simulink model "FINAL_FULL_CONTROLLER"  (R2023b)
settings: Solver=VariableStepAuto  StartTime=0.0  StopTime=10  MaxStep=1e-2  RelTol=1e-6
values from neighbouring files (symbols this model uses):
  cq = -rho*(pi*re^2)*(re^2)*Cq    (= -5.82688103164e-07)    [PARAMETRI_DRONE.m]
  Cq = 0.002508    [PARAMETRI_DRONE.m]
  ct = rho*(pi*re^2)*(re^2)*Ct    (= 3.66666014519e-06)    [PARAMETRI_DRONE.m]
  Ct = 0.015782    [PARAMETRI_DRONE.m]
  dx = 0.035/(2*sqrt(2))    [PARAMETRI_DRONE.m]
  dy = 0.035/(2*sqrt(2))    [PARAMETRI_DRONE.m]
  g = 9.81    [PARAMETRI_DRONE.m]
  I = Inertial_Matrix_DART(m1, m2, m3, m4, m, d1, d2, d3, d4, d5, dx, dy, r, h, a1, b1, c1, a2, b2, c2, a3, b3, c3, a4, b4, c4)    [PARAMETRI_DRONE.m]
  m = 0.055    [PARAMETRI_DRONE.m]
  m1 = 0.135    [PARAMETRI_DRONE.m]
  m2 = 0.602    [PARAMETRI_DRONE.m]
  m3 = 0.228    [PARAMETRI_DRONE.m]
  m4 = 0.055    [PARAMETRI_DRONE.m]
  re = 0.0889    [PARAMETRI_DRONE.m]
  wmax = RPMmax*(2*pi)/60    (= 2350.85378268)    [PARAMETRI_DRONE.m]
libraries: slpidlib x9, simulink x4, shared6dof x1, aerolibpropulsion2 x1, dspinverses x1
(part 1 of 2)
settings Model: Creator=elisa  LastModifiedBy=elisa
settings DebuggingCC: ParameterOverflowMsg=none  ParameterUnderflowMsg=error

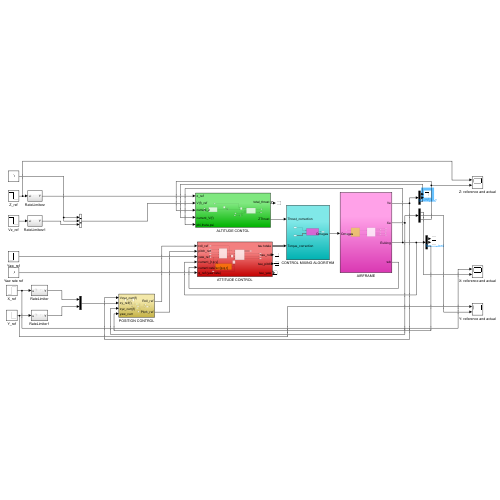
[thumbnail: Simulink's stored preview of the top-level diagram]
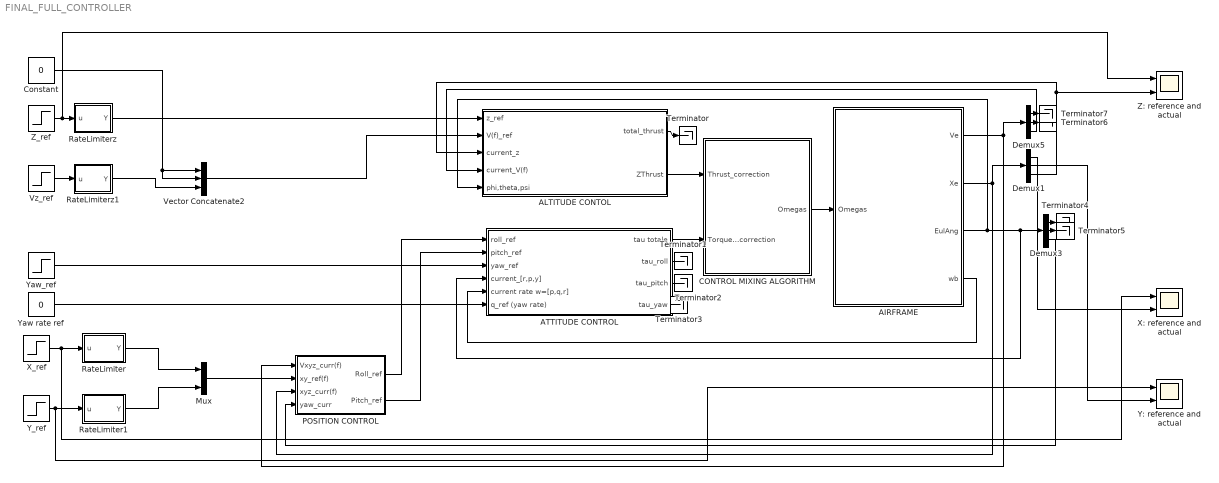
== system FINAL_FULL_CONTROLLER ==
  AIRFRAME : Subsystem
  ALTITUDE CONTOL : Subsystem
  ATTITUDE CONTROL : Subsystem
  CONTROL MIXING ALGORITHM : Subsystem
  Constant : Constant  Value=0
  Demux1 : Demux  Outputs=3
  Demux3 : Demux  Outputs=3
  Demux5 : Demux  Outputs=3
  Mux : Mux  Inputs=2
  POSITION CONTROL : Subsystem
  RateLimiter : Subsystem
  RateLimiter1 : Subsystem
  RateLimiterz : Subsystem
  RateLimiterz1 : Subsystem
  Terminator{,1..7} (8 alike) : Terminator
  Vector Concatenate2 : Concatenate  NumInputs=3
  Vz_ref : Step  After=-1  SampleTime=0
  X: reference and actual : Scope  NumInputPorts=2
  X_ref : Step  Time=2  After=0.5  SampleTime=0
  Y: reference and actual : Scope  NumInputPorts=2
  Y_ref : Step  Time=5  After=-0.2  SampleTime=0
  Yaw rate ref : Constant  Value=0
  Yaw_ref : Step  Time=6  After=pi/4  SampleTime=0
  Z: reference and actual : Scope  NumInputPorts=2
  Z_ref : Step  After=-1  SampleTime=0
  wires:
  Yaw_ref/1 -> ATTITUDE CONTROL/3(yaw_ref)
  Constant/1 -> Vector Concatenate2/1, Vector Concatenate2/2
  Yaw rate ref/1 -> ATTITUDE CONTROL/6(q_ref (yaw rate))
  AIRFRAME/4(wb) -> ATTITUDE CONTROL/5(current rate w=[p,q,r])
  AIRFRAME/2(Xe) -> POSITION CONTROL/3(xyz_curr(f)), Demux1/1
  ALTITUDE CONTOL/2(ZThrust) -> CONTROL MIXING ALGORITHM/1(Thrust_correction)
  ATTITUDE CONTROL/1(tau totale) -> CONTROL MIXING ALGORITHM/2(Torque_correction)
  Demux3/3 -> POSITION CONTROL/4(yaw_curr)
  AIRFRAME/1(Ve) -> POSITION CONTROL/1(Vxyz_curr(f)), Demux5/1
  POSITION CONTROL/1(Roll_ref) -> ATTITUDE CONTROL/1(roll_ref)
  X_ref/1 -> X: reference and actual/1, RateLimiter/1(u)
  RateLimiter/1(Y) -> Mux/1
  Y_ref/1 -> Y: reference and actual/1, RateLimiter1/1(u)
  RateLimiter1/1(Y) -> Mux/2
  Z_ref/1 -> Z: reference and actual/1, RateLimiterz/1(u)
  Vz_ref/1 -> RateLimiterz1/1(u)
  RateLimiterz1/1(Y) -> Vector Concatenate2/3
  RateLimiterz/1(Y) -> ALTITUDE CONTOL/1(z_ref)
  Vector Concatenate2/1 -> ALTITUDE CONTOL/2(V(f)_ref)
  Demux1/3 -> ALTITUDE CONTOL/3(current_z), Z: reference and actual/2
  Demux5/3 -> ALTITUDE CONTOL/4(current_V(f))
  AIRFRAME/3(EulAng) -> Demux3/1, ATTITUDE CONTROL/4(current_[r,p,y]), ALTITUDE CONTOL/5(phi,theta,psi)
  Mux/1 -> POSITION CONTROL/2(xy_ref(f))
  POSITION CONTROL/2(Pitch_ref) -> ATTITUDE CONTROL/2(pitch_ref)
  ATTITUDE CONTROL/2(tau_roll) -> Terminator1/1
  ATTITUDE CONTROL/3(tau_pitch) -> Terminator2/1
  ALTITUDE CONTOL/1(total_thrust) -> Terminator/1
  CONTROL MIXING ALGORITHM/1(Omegas) -> AIRFRAME/1(Omegas)
  Demux1/1 -> X: reference and actual/2
  Demux1/2 -> Y: reference and actual/2
  Demux3/1 -> Terminator4/1
  Demux3/2 -> Terminator5/1
  Demux5/2 -> Terminator6/1
  Demux5/1 -> Terminator7/1

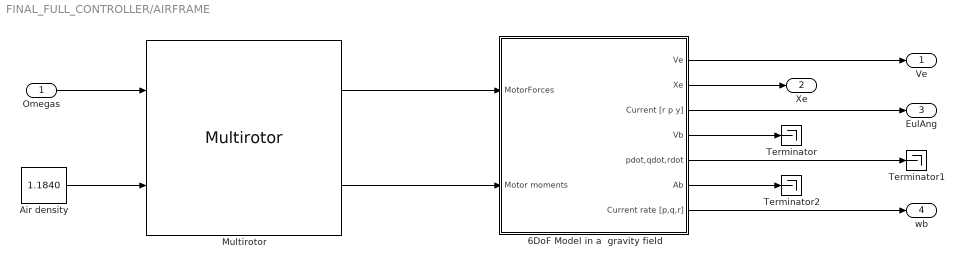
== system FINAL_FULL_CONTROLLER/AIRFRAME ==
  Omegas : Inport
  6DoF Model in a  gravity field : Subsystem
  Air density : Constant  Value=1.1840
  Multirotor : aerolibpropulsion2/Multirotor  units=Metric (MKS)  modelMode=Without flap effects  blockSelect=Multiple  config=Quadcopter X  Nr=4  l=sqrt(2)*dx  h=h  Arm=[0.0441234631460406 0.0441234631460406 -0.0441234631460406 -0.0441234631460406;-0.0441234631460406 0.0441234631460406 0.0441234631460406 -0.0441234631460406;-0.0159 -0.0159 -0.0159 -0.0159]  Nb=2  CTcheck=off  CT=Ct  CQ=Cq  CTout=off  R=re  c=0.0080  e=0  clalpha=5.5  gamma=0.6051  twistType=Linear  theta0=0.2548  theta1=-0.1361  thetaTip=0.1018  Vb=[0;0;0]  pqr=[0;0;0]
      settings: LibrarySourceBlock=aerolibrotor/Rotor
  Terminator : Terminator
  Terminator1 : Terminator
  Terminator2 : Terminator
  Ve : Outport
  Xe : Outport  Port=2
  EulAng : Outport  Port=3
  wb : Outport  Port=4
  wires:
  6DoF Model in a  gravity field/4(Vb) -> Terminator/1
  6DoF Model in a  gravity field/6(Ab) -> Terminator2/1
  6DoF Model in a  gravity field/5(pdot,qdot,rdot) -> Terminator1/1
  6DoF Model in a  gravity field/1(Ve) -> Ve/1
  6DoF Model in a  gravity field/2(Xe) -> Xe/1
  6DoF Model in a  gravity field/3(Current [r p y]) -> EulAng/1
  6DoF Model in a  gravity field/7(Current rate [p,q,r]) -> wb/1
  Multirotor/1 -> 6DoF Model in a  gravity field/1(MotorForces)
  Multirotor/2 -> 6DoF Model in a  gravity field/2(Motor moments)
  Omegas/1 -> Multirotor/1
  Air density/1 -> Multirotor/2

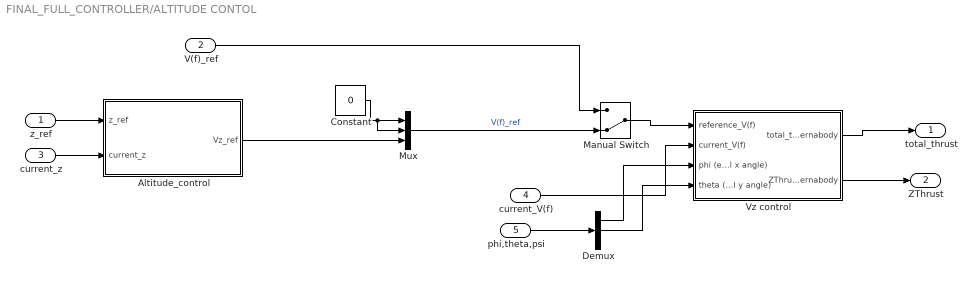
== system FINAL_FULL_CONTROLLER/ALTITUDE CONTOL ==
  z_ref : Inport
  V(f)_ref : Inport  Port=2
  current_z : Inport  Port=3
  current_V(f) : Inport  Port=4
  phi,theta,psi : Inport  Port=5
  Altitude_control : Subsystem
  Constant : Constant  Value=0
  Demux : Demux  Outputs=3
  Manual Switch : ManualSwitch  CurrentSetting=0
  Mux : Mux  Inputs=3
  Vz control : Subsystem
  total_thrust : Outport
  ZThrust : Outport  Port=2
  wires:
  current_V(f)/1 -> Vz control/2(current_V(f))
  z_ref/1 -> Altitude_control/1(z_ref)
  current_z/1 -> Altitude_control/2(current_z)
  Manual Switch/1 -> Vz control/1(reference_V(f))
  Vz control/1(total_thrust_ternabody) -> total_thrust/1
  Vz control/2(ZThrust_ternabody) -> ZThrust/1
  Mux/1 -> Manual Switch/2  "V(f)_ref"
  Altitude_control/1(Vz_ref) -> Mux/3
  Constant/1 -> Mux/2, Mux/1
  V(f)_ref/1 -> Manual Switch/1
  phi,theta,psi/1 -> Demux/1
  Demux/1 -> Vz control/3(phi (eul x angle))
  Demux/2 -> Vz control/4(theta (eul y angle))

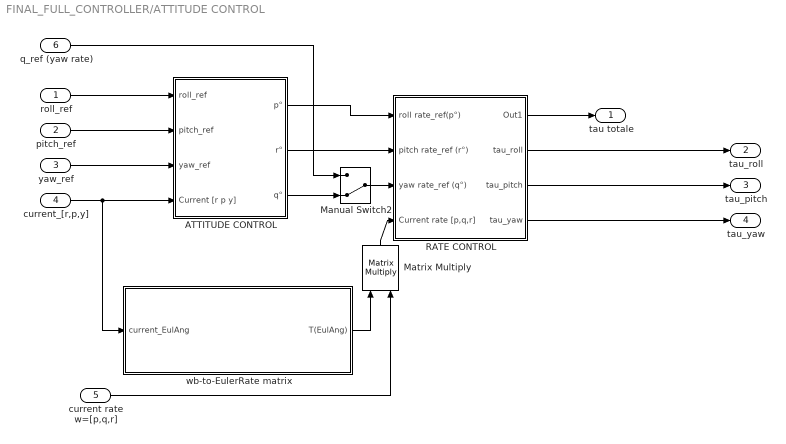
== system FINAL_FULL_CONTROLLER/ATTITUDE CONTROL ==
  roll_ref : Inport
  pitch_ref : Inport  Port=2
  yaw_ref : Inport  Port=3
  current_[r,p,y] : Inport  Port=4
  current rate w=[p,q,r] : Inport  Port=5
  q_ref (yaw rate) : Inport  Port=6
  ATTITUDE CONTROL : Subsystem
  Manual Switch2 : ManualSwitch  CurrentSetting=0
  Matrix Multiply : Product  Multiplication=Matrix(*)
  RATE CONTROL : Subsystem
  wb-to-EulerRate matrix : Subsystem
  tau totale : Outport
  tau_roll : Outport  Port=2
  tau_pitch : Outport  Port=3
  tau_yaw : Outport  Port=4
  wires:
  pitch_ref/1 -> ATTITUDE CONTROL/2(pitch_ref)
  roll_ref/1 -> ATTITUDE CONTROL/1(roll_ref)
  yaw_ref/1 -> ATTITUDE CONTROL/3(yaw_ref)
  current_[r,p,y]/1 -> wb-to-EulerRate matrix/1(current_EulAng), ATTITUDE CONTROL/4(Current [r p y])
  RATE CONTROL/1(Out1) -> tau totale/1
  ATTITUDE CONTROL/2(r°) -> RATE CONTROL/2(pitch rate_ref (r°))
  Manual Switch2/1 -> RATE CONTROL/3(yaw rate_ref (q°))
  ATTITUDE CONTROL/1(p°) -> RATE CONTROL/1(" roll rate_ref(p°)")
  q_ref (yaw rate)/1 -> Manual Switch2/1
  ATTITUDE CONTROL/3(q°) -> Manual Switch2/2
  RATE CONTROL/3(tau_pitch) -> tau_pitch/1
  RATE CONTROL/4(tau_yaw) -> tau_yaw/1
  RATE CONTROL/2(tau_roll) -> tau_roll/1
  current rate w=[p,q,r]/1 -> Matrix Multiply/2
  wb-to-EulerRate matrix/1(T(EulAng)) -> Matrix Multiply/1
  Matrix Multiply/1 -> RATE CONTROL/4(Current rate [p,q,r])

== system FINAL_FULL_CONTROLLER/CONTROL MIXING ALGORITHM ==
  Thrust_correction : Inport
  Torque_correction : Inport  Port=2
  Control Mixing Algorithm : Subsystem
  Omegas : Outport
  wires:
  Thrust_correction/1 -> Control Mixing Algorithm/1(Thrust)
  Torque_correction/1 -> Control Mixing Algorithm/2(Torque)
  Control Mixing Algorithm/1(Omega_vector) -> Omegas/1

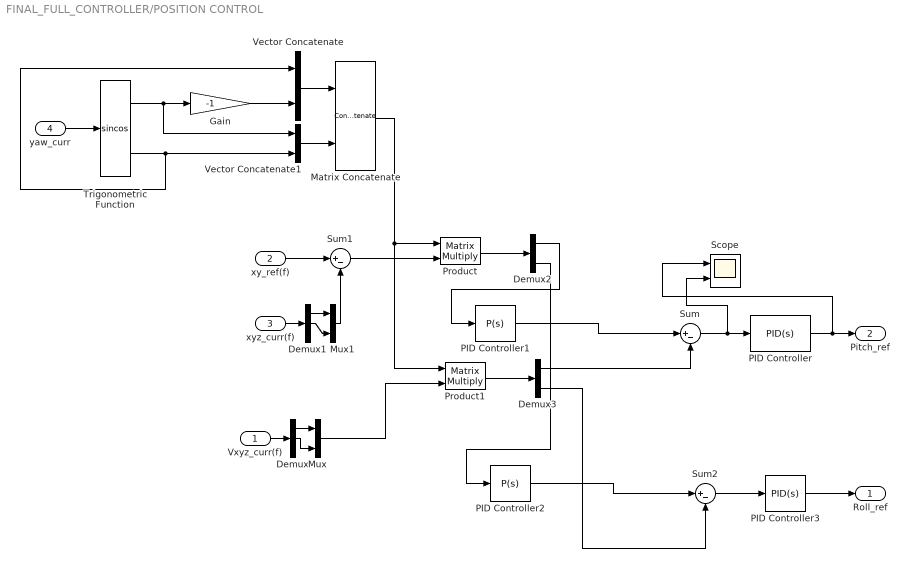
== system FINAL_FULL_CONTROLLER/POSITION CONTROL ==
  Vxyz_curr(f) : Inport
  xy_ref(f) : Inport  Port=2
  xyz_curr(f) : Inport  Port=3
  yaw_curr : Inport  Port=4
  Demux : Demux  Outputs=3
  Demux1 : Demux  Outputs=3
  Demux2 : Demux  Outputs=2
  Demux3 : Demux  Outputs=2
  Gain : Gain  Gain=-1
  Matrix Concatenate : Concatenate  Mode=Multidimensional array  ConcatenateDimension=2
  Mux : Mux  Inputs=2
  Mux1 : Mux  Inputs=2
  PID Controller : slpidlib/PID Controller  Controller=PID  Form=Parallel  TimeDomain=Continuous-time  UseExternalTs=off  SampleTime=-1  IntegratorMethod=Forward Euler  FilterMethod=Forward Euler  ControllerParametersSource=internal  P=-1.81773619393161  I=-2.23779497117918  UseKiTs=off  D=-0.196003883525991  N=1526.47988950234  UseFilter=on  TunerSelectOption=Transfer Function Based (PID Tuner App)  InitialConditionSource=internal  InitialConditionForIntegrator=0  InitialConditionForFilter=0  DifferentiatorICPrevScaledInput=0  ExternalReset=none  TrackingMode=off  Kt=1  LimitOutput=on  SatLimitsSource=internal  UpperSaturationLimit=pi/4  LowerSaturationLimit=-pi/4  LinearizeAsGain=on  AntiWindupMode=back-calculation  Kb=3  LimitIntegrator=off  UpperIntegratorSaturationLimit=inf  LowerIntegratorSaturationLimit=-inf  POutMin=[]  POutMax=[]  IOutMin=[]  IOutMax=[]  DOutMin=[]  DOutMax=[]  NOutMin=[]  NOutMax=[]  SumOutMin=[]  SumOutMax=[]  SaturationOutMin=[]  SaturationOutMax=[]  PParamMin=[]  PParamMax=[]  IParamMin=[]  IParamMax=[]  DParamMin=[]  DParamMax=[]  NParamMin=[]  NParamMax=[]  KbParamMin=[]  KbParamMax=[]  KtParamMin=[]  KtParamMax=[]  KbOutMin=[]  KbOutMax=[]  KtOutMin=[]  KtOutMax=[]  IntegratorOutMin=[]  IntegratorOutMax=[]  FilterOutMin=[]  FilterOutMax=[]  SumI1OutMin=[]  SumI1OutMax=[]  SumI2OutMin=[]  SumI2OutMax=[]  SumI3OutMin=[]  SumI3OutMax=[]  SumI4OutMin=[]  SumI4OutMax=[]  SumDOutMin=[]  SumDOutMax=[]  DifferentiatorOutMin=[]  DifferentiatorOutMax=[]  FilterDiffOutCoefMin=[]  FilterDiffOutCoefMax=[]  ReciprocalOutMin=[]  ReciprocalOutMax=[]  SumDenOutMin=[]  SumDenOutMax=[]  SumNumOutMin=[]  SumNumOutMax=[]  DivideOutMin=[]  DivideOutMax=[]  UdiffTsProdOutMin=[]  UdiffTsProdOutMax=[]  NTsProdOutMin=[]  NTsProdOutMax=[]  UintegralTsProdOutMin=[]  UintegralTsProdOutMax=[]  UngainTsProdOutMin=[]  UngainTsProdOutMax=[]  ClampingZeroOutDataTypeStr=Inherit: Inherit via back propagation  ClampingZeroOutMin=[]  ClampingZeroOutMax=[]  FilterDenConstantOutDataTypeStr=Inherit: Inherit via back propagation  FilterDenConstantOutMin=[]  FilterDenConstantOutMax=[]  PCopyOutDataTypeStr=Inherit: Inherit via back propagation  PCopyOutMin=[]  PCopyOutMax=[]  NCopyOutDataTypeStr=Inherit: Inherit via back propagation  NCopyOutMin=[]  NCopyOutMax=[]  IntegratorContinuousStateAttributes=''  IntegratorStateMustResolveToSignalObject=off  IntegratorRTWStateStorageClass=Auto  FilterContinuousStateAttributes=''  FilterStateMustResolveToSignalObject=off  FilterRTWStateStorageClass=Auto  ParallelPVariant=InternalParameters  IdealPVariant=Disabled  IVariant=InternalParameters  DVariant=InternalParameters  IntegratorVariant=Continuous  SatVariant=Enabled  AWVariant=BackCalculation  PCopyVariant=Disabled  TRVariant=Disabled  FdbkBlocksVariant=Forward  IdealPFdbkVariant=Disabled  SatFdbkVariant=Disabled  DerivativeFilterVariant=ContFilter  NVariant=InternalParameters  NCopyVariant=Disabled  FilterICVariant=InternalICsFilter  IntegratorICVariant=InternalICs  ExternalResetVariant=Disabled  TRSumVariant=Passthrough  SumFdbkVariant=Disabled  SumVariant=Sum_PID  TsampFilterVariant=InternalTs  TsampNgainVariant=Passthrough  TsampIntegralVariant=Disabled_SignalSpec  ExternalSaturationOutDataTypeStr=Inherit: Same as second input
  PID Controller1 : slpidlib/PID Controller  Controller=P  Form=Parallel  TimeDomain=Continuous-time  UseExternalTs=off  SampleTime=-1  IntegratorMethod=Forward Euler  FilterMethod=Forward Euler  ControllerParametersSource=internal  P=6.73453826135935  I=1  UseKiTs=off  D=0  N=100  UseFilter=on  TunerSelectOption=Transfer Function Based (PID Tuner App)  InitialConditionSource=internal  InitialConditionForIntegrator=0  InitialConditionForFilter=0  DifferentiatorICPrevScaledInput=0  ExternalReset=none  TrackingMode=off  Kt=1  LimitOutput=off  SatLimitsSource=internal  UpperSaturationLimit=inf  LowerSaturationLimit=-inf  LinearizeAsGain=on  AntiWindupMode=none  Kb=1  LimitIntegrator=off  UpperIntegratorSaturationLimit=inf  LowerIntegratorSaturationLimit=-inf  POutMin=[]  POutMax=[]  IOutMin=[]  IOutMax=[]  DOutMin=[]  DOutMax=[]  NOutMin=[]  NOutMax=[]  SumOutMin=[]  SumOutMax=[]  SaturationOutMin=[]  SaturationOutMax=[]  PParamMin=[]  PParamMax=[]  IParamMin=[]  IParamMax=[]  DParamMin=[]  DParamMax=[]  NParamMin=[]  NParamMax=[]  KbParamMin=[]  KbParamMax=[]  KtParamMin=[]  KtParamMax=[]  KbOutMin=[]  KbOutMax=[]  KtOutMin=[]  KtOutMax=[]  IntegratorOutMin=[]  IntegratorOutMax=[]  FilterOutMin=[]  FilterOutMax=[]  SumI1OutMin=[]  SumI1OutMax=[]  SumI2OutMin=[]  SumI2OutMax=[]  SumI3OutMin=[]  SumI3OutMax=[]  SumI4OutMin=[]  SumI4OutMax=[]  SumDOutMin=[]  SumDOutMax=[]  DifferentiatorOutMin=[]  DifferentiatorOutMax=[]  FilterDiffOutCoefMin=[]  FilterDiffOutCoefMax=[]  ReciprocalOutMin=[]  ReciprocalOutMax=[]  SumDenOutMin=[]  SumDenOutMax=[]  SumNumOutMin=[]  SumNumOutMax=[]  DivideOutMin=[]  DivideOutMax=[]  UdiffTsProdOutMin=[]  UdiffTsProdOutMax=[]  NTsProdOutMin=[]  NTsProdOutMax=[]  UintegralTsProdOutMin=[]  UintegralTsProdOutMax=[]  UngainTsProdOutMin=[]  UngainTsProdOutMax=[]  ClampingZeroOutDataTypeStr=Inherit: Inherit via back propagation  ClampingZeroOutMin=[]  ClampingZeroOutMax=[]  FilterDenConstantOutDataTypeStr=Inherit: Inherit via back propagation  FilterDenConstantOutMin=[]  FilterDenConstantOutMax=[]  PCopyOutDataTypeStr=Inherit: Inherit via back propagation  PCopyOutMin=[]  PCopyOutMax=[]  NCopyOutDataTypeStr=Inherit: Inherit via back propagation  NCopyOutMin=[]  NCopyOutMax=[]  IntegratorContinuousStateAttributes=''  IntegratorStateMustResolveToSignalObject=off  IntegratorRTWStateStorageClass=Auto  FilterContinuousStateAttributes=''  FilterStateMustResolveToSignalObject=off  FilterRTWStateStorageClass=Auto  ParallelPVariant=InternalParameters  IdealPVariant=Disabled  IVariant=Disabled  DVariant=Disabled  IntegratorVariant=Disabled  SatVariant=Disabled  AWVariant=Disabled  PCopyVariant=Disabled  TRVariant=Disabled  FdbkBlocksVariant=Forward  IdealPFdbkVariant=Disabled  SatFdbkVariant=Disabled  DerivativeFilterVariant=Disabled  NVariant=Disabled  NCopyVariant=Disabled_SignalSpec  FilterICVariant=Disabled  IntegratorICVariant=Disabled  ExternalResetVariant=Disabled  TRSumVariant=Passthrough  SumFdbkVariant=Disabled  SumVariant=Passthrough_P  TsampFilterVariant=InternalTs  TsampNgainVariant=Passthrough  TsampIntegralVariant=Disabled_SignalSpec  ExternalSaturationOutDataTypeStr=Inherit: Same as second input
  PID Controller2 : slpidlib/PID Controller  Controller=P  Form=Parallel  TimeDomain=Continuous-time  UseExternalTs=off  SampleTime=-1  IntegratorMethod=Forward Euler  FilterMethod=Forward Euler  ControllerParametersSource=internal  P=6.91764423663116  I=1  UseKiTs=off  D=0  N=100  UseFilter=on  TunerSelectOption=Transfer Function Based (PID Tuner App)  InitialConditionSource=internal  InitialConditionForIntegrator=0  InitialConditionForFilter=0  DifferentiatorICPrevScaledInput=0  ExternalReset=none  TrackingMode=off  Kt=1  LimitOutput=off  SatLimitsSource=internal  UpperSaturationLimit=inf  LowerSaturationLimit=-inf  LinearizeAsGain=on  AntiWindupMode=none  Kb=1  LimitIntegrator=off  UpperIntegratorSaturationLimit=inf  LowerIntegratorSaturationLimit=-inf  POutMin=[]  POutMax=[]  IOutMin=[]  IOutMax=[]  DOutMin=[]  DOutMax=[]  NOutMin=[]  NOutMax=[]  SumOutMin=[]  SumOutMax=[]  SaturationOutMin=[]  SaturationOutMax=[]  PParamMin=[]  PParamMax=[]  IParamMin=[]  IParamMax=[]  DParamMin=[]  DParamMax=[]  NParamMin=[]  NParamMax=[]  KbParamMin=[]  KbParamMax=[]  KtParamMin=[]  KtParamMax=[]  KbOutMin=[]  KbOutMax=[]  KtOutMin=[]  KtOutMax=[]  IntegratorOutMin=[]  IntegratorOutMax=[]  FilterOutMin=[]  FilterOutMax=[]  SumI1OutMin=[]  SumI1OutMax=[]  SumI2OutMin=[]  SumI2OutMax=[]  SumI3OutMin=[]  SumI3OutMax=[]  SumI4OutMin=[]  SumI4OutMax=[]  SumDOutMin=[]  SumDOutMax=[]  DifferentiatorOutMin=[]  DifferentiatorOutMax=[]  FilterDiffOutCoefMin=[]  FilterDiffOutCoefMax=[]  ReciprocalOutMin=[]  ReciprocalOutMax=[]  SumDenOutMin=[]  SumDenOutMax=[]  SumNumOutMin=[]  SumNumOutMax=[]  DivideOutMin=[]  DivideOutMax=[]  UdiffTsProdOutMin=[]  UdiffTsProdOutMax=[]  NTsProdOutMin=[]  NTsProdOutMax=[]  UintegralTsProdOutMin=[]  UintegralTsProdOutMax=[]  UngainTsProdOutMin=[]  UngainTsProdOutMax=[]  ClampingZeroOutDataTypeStr=Inherit: Inherit via back propagation  ClampingZeroOutMin=[]  ClampingZeroOutMax=[]  FilterDenConstantOutDataTypeStr=Inherit: Inherit via back propagation  FilterDenConstantOutMin=[]  FilterDenConstantOutMax=[]  PCopyOutDataTypeStr=Inherit: Inherit via back propagation  PCopyOutMin=[]  PCopyOutMax=[]  NCopyOutDataTypeStr=Inherit: Inherit via back propagation  NCopyOutMin=[]  NCopyOutMax=[]  IntegratorContinuousStateAttributes=''  IntegratorStateMustResolveToSignalObject=off  IntegratorRTWStateStorageClass=Auto  FilterContinuousStateAttributes=''  FilterStateMustResolveToSignalObject=off  FilterRTWStateStorageClass=Auto  ParallelPVariant=InternalParameters  IdealPVariant=Disabled  IVariant=Disabled  DVariant=Disabled  IntegratorVariant=Disabled  SatVariant=Disabled  AWVariant=Disabled  PCopyVariant=Disabled  TRVariant=Disabled  FdbkBlocksVariant=Forward  IdealPFdbkVariant=Disabled  SatFdbkVariant=Disabled  DerivativeFilterVariant=Disabled  NVariant=Disabled  NCopyVariant=Disabled_SignalSpec  FilterICVariant=Disabled  IntegratorICVariant=Disabled  ExternalResetVariant=Disabled  TRSumVariant=Passthrough  SumFdbkVariant=Disabled  SumVariant=Passthrough_P  TsampFilterVariant=InternalTs  TsampNgainVariant=Passthrough  TsampIntegralVariant=Disabled_SignalSpec  ExternalSaturationOutDataTypeStr=Inherit: Same as second input
  PID Controller3 : slpidlib/PID Controller  Controller=PID  Form=Parallel  TimeDomain=Continuous-time  UseExternalTs=off  SampleTime=-1  IntegratorMethod=Forward Euler  FilterMethod=Forward Euler  ControllerParametersSource=internal  P=1.72614492788019  I=2.41380700470898  UseKiTs=off  D=0.203044940466474  N=1625.25083963237  UseFilter=on  TunerSelectOption=Transfer Function Based (PID Tuner App)  InitialConditionSource=internal  InitialConditionForIntegrator=0  InitialConditionForFilter=0  DifferentiatorICPrevScaledInput=0  ExternalReset=none  TrackingMode=off  Kt=1  LimitOutput=on  SatLimitsSource=internal  UpperSaturationLimit=pi/4  LowerSaturationLimit=-pi/4  LinearizeAsGain=on  AntiWindupMode=back-calculation  Kb=3  LimitIntegrator=off  UpperIntegratorSaturationLimit=inf  LowerIntegratorSaturationLimit=-inf  POutMin=[]  POutMax=[]  IOutMin=[]  IOutMax=[]  DOutMin=[]  DOutMax=[]  NOutMin=[]  NOutMax=[]  SumOutMin=[]  SumOutMax=[]  SaturationOutMin=[]  SaturationOutMax=[]  PParamMin=[]  PParamMax=[]  IParamMin=[]  IParamMax=[]  DParamMin=[]  DParamMax=[]  NParamMin=[]  NParamMax=[]  KbParamMin=[]  KbParamMax=[]  KtParamMin=[]  KtParamMax=[]  KbOutMin=[]  KbOutMax=[]  KtOutMin=[]  KtOutMax=[]  IntegratorOutMin=[]  IntegratorOutMax=[]  FilterOutMin=[]  FilterOutMax=[]  SumI1OutMin=[]  SumI1OutMax=[]  SumI2OutMin=[]  SumI2OutMax=[]  SumI3OutMin=[]  SumI3OutMax=[]  SumI4OutMin=[]  SumI4OutMax=[]  SumDOutMin=[]  SumDOutMax=[]  DifferentiatorOutMin=[]  DifferentiatorOutMax=[]  FilterDiffOutCoefMin=[]  FilterDiffOutCoefMax=[]  ReciprocalOutMin=[]  ReciprocalOutMax=[]  SumDenOutMin=[]  SumDenOutMax=[]  SumNumOutMin=[]  SumNumOutMax=[]  DivideOutMin=[]  DivideOutMax=[]  UdiffTsProdOutMin=[]  UdiffTsProdOutMax=[]  NTsProdOutMin=[]  NTsProdOutMax=[]  UintegralTsProdOutMin=[]  UintegralTsProdOutMax=[]  UngainTsProdOutMin=[]  UngainTsProdOutMax=[]  ClampingZeroOutDataTypeStr=Inherit: Inherit via back propagation  ClampingZeroOutMin=[]  ClampingZeroOutMax=[]  FilterDenConstantOutDataTypeStr=Inherit: Inherit via back propagation  FilterDenConstantOutMin=[]  FilterDenConstantOutMax=[]  PCopyOutDataTypeStr=Inherit: Inherit via back propagation  PCopyOutMin=[]  PCopyOutMax=[]  NCopyOutDataTypeStr=Inherit: Inherit via back propagation  NCopyOutMin=[]  NCopyOutMax=[]  IntegratorContinuousStateAttributes=''  IntegratorStateMustResolveToSignalObject=off  IntegratorRTWStateStorageClass=Auto  FilterContinuousStateAttributes=''  FilterStateMustResolveToSignalObject=off  FilterRTWStateStorageClass=Auto  ParallelPVariant=InternalParameters  IdealPVariant=Disabled  IVariant=InternalParameters  DVariant=InternalParameters  IntegratorVariant=Continuous  SatVariant=Enabled  AWVariant=BackCalculation  PCopyVariant=Disabled  TRVariant=Disabled  FdbkBlocksVariant=Forward  IdealPFdbkVariant=Disabled  SatFdbkVariant=Disabled  DerivativeFilterVariant=ContFilter  NVariant=InternalParameters  NCopyVariant=Disabled  FilterICVariant=InternalICsFilter  IntegratorICVariant=InternalICs  ExternalResetVariant=Disabled  TRSumVariant=Passthrough  SumFdbkVariant=Disabled  SumVariant=Sum_PID  TsampFilterVariant=InternalTs  TsampNgainVariant=Passthrough  TsampIntegralVariant=Disabled_SignalSpec  ExternalSaturationOutDataTypeStr=Inherit: Same as second input
  Product : Product  Multiplication=Matrix(*)  OutDataTypeStr=single  RndMeth=Zero
  Product1 : Product  Multiplication=Matrix(*)  OutDataTypeStr=single  RndMeth=Zero
  Scope : Scope  NumInputPorts=2
  Sum : Sum  Inputs=|+-
  Sum1 : Sum  Inputs=|+-
  Sum2 : Sum  Inputs=|+-
  Trigonometric Function : Trigonometry  Operator=sincos
  Vector Concatenate : Concatenate
  Vector Concatenate1 : Concatenate
  Roll_ref : Outport
  Pitch_ref : Outport  Port=2
  wires:
  PID Controller/1 -> Scope/1, Pitch_ref/1
  Vxyz_curr(f)/1 -> Demux/1
  xy_ref(f)/1 -> Sum1/1
  xyz_curr(f)/1 -> Demux1/1
  Gain/1 -> Vector Concatenate/2
  yaw_curr/1 -> Trigonometric Function/1
  Matrix Concatenate/1 -> Product1/1, Product/1
  Vector Concatenate1/1 -> Matrix Concatenate/2
  Trigonometric Function/1 -> Gain/1, Vector Concatenate1/1
  Vector Concatenate/1 -> Matrix Concatenate/1
  Trigonometric Function/2 -> Vector Concatenate1/2, Vector Concatenate/1
  Sum1/1 -> Product/2
  Product/1 -> Demux2/1
  Demux/1 -> Mux/1
  Demux/2 -> Mux/2
  Mux/1 -> Product1/2
  Product1/1 -> Demux3/1
  Demux3/1 -> Sum/2
  Sum/1 -> Scope/2, PID Controller/1
  Demux2/1 -> PID Controller1/1
  PID Controller1/1 -> Sum/1
  Demux1/1 -> Mux1/1
  Demux1/2 -> Mux1/2
  Mux1/1 -> Sum1/2
  PID Controller2/1 -> Sum2/1
  Sum2/1 -> PID Controller3/1
  Demux2/2 -> PID Controller2/1
  Demux3/2 -> Sum2/2
  PID Controller3/1 -> Roll_ref/1

== system FINAL_FULL_CONTROLLER/RateLimiter ==
  u : Inport
  Constant2 : Constant  Value=-0.25
  Constant4 : Constant  Value=0.25
  Rate Limiter Dynamic1 : simulink/Discontinuities/Rate Limiter Dynamic
  Y : Outport
  wires:
  Constant2/1 -> Rate Limiter Dynamic1/3
  Rate Limiter Dynamic1/1 -> Y/1
  Constant4/1 -> Rate Limiter Dynamic1/1
  u/1 -> Rate Limiter Dynamic1/2

== system FINAL_FULL_CONTROLLER/RateLimiter1 ==
  u : Inport
  Constant2 : Constant  Value=-0.25
  Constant4 : Constant  Value=0.25
  Rate Limiter Dynamic1 : simulink/Discontinuities/Rate Limiter Dynamic
  Y : Outport
  wires:
  Constant2/1 -> Rate Limiter Dynamic1/3
  Rate Limiter Dynamic1/1 -> Y/1
  Constant4/1 -> Rate Limiter Dynamic1/1
  u/1 -> Rate Limiter Dynamic1/2

== system FINAL_FULL_CONTROLLER/RateLimiterz ==
  u : Inport
  Constant1 : Constant  Value=2
  Constant5 : Constant  Value=-2
  Rate Limiter Dynamic3 : simulink/Discontinuities/Rate Limiter Dynamic
  Y : Outport
  wires:
  Rate Limiter Dynamic3/1 -> Y/1
  Constant5/1 -> Rate Limiter Dynamic3/3
  Constant1/1 -> Rate Limiter Dynamic3/1
  u/1 -> Rate Limiter Dynamic3/2

== system FINAL_FULL_CONTROLLER/RateLimiterz1 ==
  u : Inport
  Constant1 : Constant  Value=2
  Constant5 : Constant  Value=-2
  Rate Limiter Dynamic3 : simulink/Discontinuities/Rate Limiter Dynamic
  Y : Outport
  wires:
  Rate Limiter Dynamic3/1 -> Y/1
  Constant5/1 -> Rate Limiter Dynamic3/3
  Constant1/1 -> Rate Limiter Dynamic3/1
  u/1 -> Rate Limiter Dynamic3/2

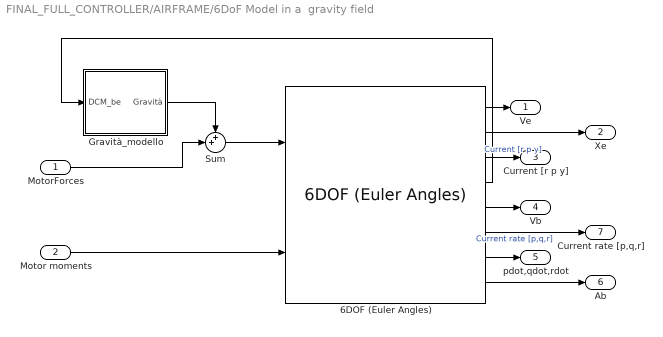
== system FINAL_FULL_CONTROLLER/AIRFRAME/6DoF Model in a  gravity field ==
  MotorForces : Inport
  Motor moments : Inport  Port=2
  6DOF (Euler Angles) : shared6dof/6DOF (Euler Angles)  units=Metric (MKS)  mtype=Fixed  rep=Euler Angles  xme_0=[0 0 0]  Vm_0=[0 0 0]  eul_0=[0 0 0]  pm_0=[0 0 0]  mass_0=m1+m2+m3+m4+4*m  mass_e=0.5  mass_f=2.0  inertia=I  inertia_e=eye(3)  inertia_f=2*eye(3)  k_quat=1.0  vre_flag=on  abi_flag=off  aMode=0  xme_statename=''  Vm_statename=''  eul_statename=''  quat_statename=''  pm_statename=''  mass_statename=''
  Gravità_modello : Subsystem
  Sum : Sum  Inputs=++|
  Ve : Outport
  Xe : Outport  Port=2
  Current [r p y] : Outport  Port=3
  Vb : Outport  Port=4
  pdot,qdot,rdot : Outport  Port=5
  Ab : Outport  Port=6
  Current rate [p,q,r] : Outport  Port=7
  wires:
  6DOF (Euler Angles)/2 -> Xe/1
  6DOF (Euler Angles)/3 -> Current [r p y]/1  "Current [r p y]"
  Sum/1 -> 6DOF (Euler Angles)/1
  6DOF (Euler Angles)/7 -> pdot,qdot,rdot/1
  6DOF (Euler Angles)/4 -> Gravità_modello/1(DCM_be)
  Motor moments/1 -> 6DOF (Euler Angles)/2
  6DOF (Euler Angles)/6 -> Current rate [p,q,r]/1  "Current rate [p,q,r]"
  6DOF (Euler Angles)/1 -> Ve/1
  6DOF (Euler Angles)/5 -> Vb/1
  6DOF (Euler Angles)/8 -> Ab/1
  MotorForces/1 -> Sum/2
  Gravità_modello/1(Gravità) -> Sum/1

== system FINAL_FULL_CONTROLLER/ALTITUDE CONTOL/Altitude_control ==
  z_ref : Inport
  current_z : Inport  Port=2
  PID Controller3 : slpidlib/PID Controller  Controller=P  Form=Parallel  TimeDomain=Continuous-time  UseExternalTs=off  SampleTime=-1  IntegratorMethod=Forward Euler  FilterMethod=Forward Euler  ControllerParametersSource=internal  P=5.6850902998465  I=1  UseKiTs=off  D=6.06699485897849  N=453.788908646381  UseFilter=on  TunerSelectOption=Transfer Function Based (PID Tuner App)  InitialConditionSource=internal  InitialConditionForIntegrator=0  InitialConditionForFilter=0  DifferentiatorICPrevScaledInput=0  ExternalReset=none  TrackingMode=off  Kt=1  LimitOutput=off  SatLimitsSource=internal  UpperSaturationLimit=inf  LowerSaturationLimit=-inf  LinearizeAsGain=on  AntiWindupMode=none  Kb=1  LimitIntegrator=off  UpperIntegratorSaturationLimit=inf  LowerIntegratorSaturationLimit=-inf  POutMin=[]  POutMax=[]  IOutMin=[]  IOutMax=[]  DOutMin=[]  DOutMax=[]  NOutMin=[]  NOutMax=[]  SumOutMin=[]  SumOutMax=[]  SaturationOutMin=[]  SaturationOutMax=[]  PParamMin=[]  PParamMax=[]  IParamMin=[]  IParamMax=[]  DParamMin=[]  DParamMax=[]  NParamMin=[]  NParamMax=[]  KbParamMin=[]  KbParamMax=[]  KtParamMin=[]  KtParamMax=[]  KbOutMin=[]  KbOutMax=[]  KtOutMin=[]  KtOutMax=[]  IntegratorOutMin=[]  IntegratorOutMax=[]  FilterOutMin=[]  FilterOutMax=[]  SumI1OutMin=[]  SumI1OutMax=[]  SumI2OutMin=[]  SumI2OutMax=[]  SumI3OutMin=[]  SumI3OutMax=[]  SumI4OutMin=[]  SumI4OutMax=[]  SumDOutMin=[]  SumDOutMax=[]  DifferentiatorOutMin=[]  DifferentiatorOutMax=[]  FilterDiffOutCoefMin=[]  FilterDiffOutCoefMax=[]  ReciprocalOutMin=[]  ReciprocalOutMax=[]  SumDenOutMin=[]  SumDenOutMax=[]  SumNumOutMin=[]  SumNumOutMax=[]  DivideOutMin=[]  DivideOutMax=[]  UdiffTsProdOutMin=[]  UdiffTsProdOutMax=[]  NTsProdOutMin=[]  NTsProdOutMax=[]  UintegralTsProdOutMin=[]  UintegralTsProdOutMax=[]  UngainTsProdOutMin=[]  UngainTsProdOutMax=[]  ClampingZeroOutDataTypeStr=Inherit: Inherit via back propagation  ClampingZeroOutMin=[]  ClampingZeroOutMax=[]  FilterDenConstantOutDataTypeStr=Inherit: Inherit via back propagation  FilterDenConstantOutMin=[]  FilterDenConstantOutMax=[]  PCopyOutDataTypeStr=Inherit: Inherit via back propagation  PCopyOutMin=[]  PCopyOutMax=[]  NCopyOutDataTypeStr=Inherit: Inherit via back propagation  NCopyOutMin=[]  NCopyOutMax=[]  IntegratorContinuousStateAttributes=''  IntegratorStateMustResolveToSignalObject=off  IntegratorRTWStateStorageClass=Auto  FilterContinuousStateAttributes=''  FilterStateMustResolveToSignalObject=off  FilterRTWStateStorageClass=Auto  ParallelPVariant=InternalParameters  IdealPVariant=Disabled  IVariant=Disabled  DVariant=Disabled  IntegratorVariant=Disabled  SatVariant=Disabled  AWVariant=Disabled  PCopyVariant=Disabled  TRVariant=Disabled  FdbkBlocksVariant=Forward  IdealPFdbkVariant=Disabled  SatFdbkVariant=Disabled  DerivativeFilterVariant=Disabled  NVariant=Disabled  NCopyVariant=Disabled_SignalSpec  FilterICVariant=Disabled  IntegratorICVariant=Disabled  ExternalResetVariant=Disabled  TRSumVariant=Passthrough  SumFdbkVariant=Disabled  SumVariant=Passthrough_P  TsampFilterVariant=InternalTs  TsampNgainVariant=Passthrough  TsampIntegralVariant=Disabled_SignalSpec  ExternalSaturationOutDataTypeStr=Inherit: Same as second input
  Sum2 : Sum  Inputs=|+-
  Vz_ref : Outport
  wires:
  z_ref/1 -> Sum2/1
  Sum2/1 -> PID Controller3/1
  current_z/1 -> Sum2/2
  PID Controller3/1 -> Vz_ref/1  "Vz_reference"

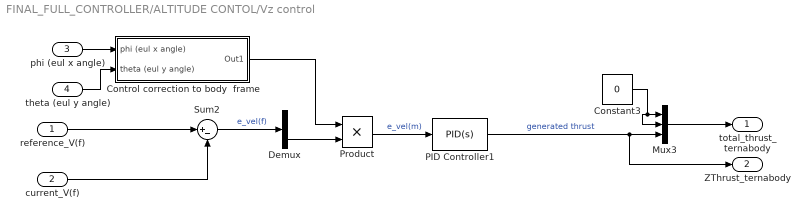
== system FINAL_FULL_CONTROLLER/ALTITUDE CONTOL/Vz control ==
  reference_V(f) : Inport
  current_V(f) : Inport  Port=2
  phi (eul x angle) : Inport  Port=3
  theta (eul y angle) : Inport  Port=4
  Constant3 : Constant  Value=0
  Control correction to body  frame : Subsystem
  Demux : Demux  Outputs=3
  Mux3 : Mux  Inputs=3
  PID Controller1 : slpidlib/PID Controller  Controller=PID  Form=Parallel  TimeDomain=Continuous-time  UseExternalTs=off  SampleTime=-1  IntegratorMethod=Forward Euler  FilterMethod=Forward Euler  ControllerParametersSource=internal  P=25.2963813497766  I=48.2492876003403  UseKiTs=off  D=-0.202447305909655  N=33.8830483713043  UseFilter=on  TunerSelectOption=Transfer Function Based (PID Tuner App)  InitialConditionSource=internal  InitialConditionForIntegrator=0  InitialConditionForFilter=0  DifferentiatorICPrevScaledInput=0  ExternalReset=none  TrackingMode=off  Kt=1  LimitOutput=on  SatLimitsSource=internal  UpperSaturationLimit=0  LowerSaturationLimit=-4*ct*wmax^2  LinearizeAsGain=on  AntiWindupMode=back-calculation  Kb=5  LimitIntegrator=off  UpperIntegratorSaturationLimit=inf  LowerIntegratorSaturationLimit=-inf  RndMeth=Simplest  POutMin=[]  POutMax=[]  IOutMin=[]  IOutMax=[]  DOutMin=[]  DOutMax=[]  NOutMin=[]  NOutMax=[]  SumOutMin=[]  SumOutMax=[]  SaturationOutMin=[]  SaturationOutMax=[]  PParamMin=[]  PParamMax=[]  IParamMin=[]  IParamMax=[]  DParamMin=[]  DParamMax=[]  NParamMin=[]  NParamMax=[]  KbParamMin=[]  KbParamMax=[]  KtParamMin=[]  KtParamMax=[]  KbOutMin=[]  KbOutMax=[]  KtOutMin=[]  KtOutMax=[]  IntegratorOutMin=[]  IntegratorOutMax=[]  FilterOutMin=[]  FilterOutMax=[]  SumI1OutMin=[]  SumI1OutMax=[]  SumI2OutMin=[]  SumI2OutMax=[]  SumI3OutMin=[]  SumI3OutMax=[]  SumI4OutMin=[]  SumI4OutMax=[]  SumDOutMin=[]  SumDOutMax=[]  DifferentiatorOutMin=[]  DifferentiatorOutMax=[]  FilterDiffOutCoefMin=[]  FilterDiffOutCoefMax=[]  ReciprocalOutMin=[]  ReciprocalOutMax=[]  SumDenOutMin=[]  SumDenOutMax=[]  SumNumOutMin=[]  SumNumOutMax=[]  DivideOutMin=[]  DivideOutMax=[]  UdiffTsProdOutMin=[]  UdiffTsProdOutMax=[]  NTsProdOutMin=[]  NTsProdOutMax=[]  UintegralTsProdOutMin=[]  UintegralTsProdOutMax=[]  UngainTsProdOutMin=[]  UngainTsProdOutMax=[]  ClampingZeroOutDataTypeStr=Inherit: Inherit via back propagation  ClampingZeroOutMin=[]  ClampingZeroOutMax=[]  FilterDenConstantOutDataTypeStr=Inherit: Inherit via back propagation  FilterDenConstantOutMin=[]  FilterDenConstantOutMax=[]  PCopyOutDataTypeStr=Inherit: Inherit via back propagation  PCopyOutMin=[]  PCopyOutMax=[]  NCopyOutDataTypeStr=Inherit: Inherit via back propagation  NCopyOutMin=[]  NCopyOutMax=[]  IntegratorContinuousStateAttributes=''  IntegratorStateMustResolveToSignalObject=off  IntegratorRTWStateStorageClass=Auto  FilterContinuousStateAttributes=''  FilterStateMustResolveToSignalObject=off  FilterRTWStateStorageClass=Auto  ParallelPVariant=InternalParameters  IdealPVariant=Disabled  IVariant=InternalParameters  DVariant=InternalParameters  IntegratorVariant=Continuous  SatVariant=Enabled  AWVariant=BackCalculation  PCopyVariant=Disabled  TRVariant=Disabled  FdbkBlocksVariant=Forward  IdealPFdbkVariant=Disabled  SatFdbkVariant=Disabled  DerivativeFilterVariant=ContFilter  NVariant=InternalParameters  NCopyVariant=Disabled  FilterICVariant=InternalICsFilter  IntegratorICVariant=InternalICs  ExternalResetVariant=Disabled  TRSumVariant=Passthrough  SumFdbkVariant=Disabled  SumVariant=Sum_PID  TsampFilterVariant=InternalTs  TsampNgainVariant=Passthrough  TsampIntegralVariant=Disabled_SignalSpec  ExternalSaturationOutDataTypeStr=Inherit: Same as second input
  Product : Product
  Sum2 : Sum  Inputs=|+-
  total_thrust_ternabody : Outport
  ZThrust_ternabody : Outport  Port=2
  wires:
  Mux3/1 -> total_thrust_ternabody/1
  Constant3/1 -> Mux3/2, Mux3/1
  reference_V(f)/1 -> Sum2/1
  current_V(f)/1 -> Sum2/2
  Sum2/1 -> Demux/1  "e_vel(f)"
  phi (eul x angle)/1 -> Control correction to body  frame/1(phi (eul x angle))
  theta (eul y angle)/1 -> Control correction to body  frame/2(theta (eul y angle))
  Control correction to body  frame/1(Out1) -> Product/1
  Product/1 -> PID Controller1/1  "e_vel(m)"
  Demux/3 -> Product/2
  PID Controller1/1 -> ZThrust_ternabody/1, Mux3/3  "generated thrust"

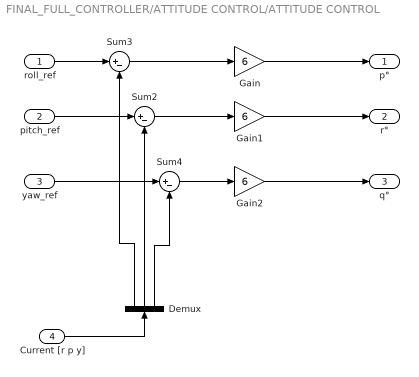
== system FINAL_FULL_CONTROLLER/ATTITUDE CONTROL/ATTITUDE CONTROL ==
  roll_ref : Inport
  pitch_ref : Inport  Port=2
  yaw_ref : Inport  Port=3
  Current [r p y] : Inport  Port=4
  Demux : Demux  Outputs=3
  Gain : Gain  Gain=6
  Gain1 : Gain  Gain=6
  Gain2 : Gain  Gain=6
  Sum2 : Sum  Inputs=|+-
  Sum3 : Sum  Inputs=|+-
  Sum4 : Sum  Inputs=|+-
  p° : Outport
  r° : Outport  Port=2
  q° : Outport  Port=3
  wires:
  Demux/1 -> Sum3/2
  Sum2/1 -> Gain1/1
  roll_ref/1 -> Sum3/1
  Demux/3 -> Sum4/2
  Gain1/1 -> r°/1
  Sum3/1 -> Gain/1
  Demux/2 -> Sum2/2
  Sum4/1 -> Gain2/1
  pitch_ref/1 -> Sum2/1
  yaw_ref/1 -> Sum4/1
  Current [r p y]/1 -> Demux/1
  Gain/1 -> p°/1
  Gain2/1 -> q°/1

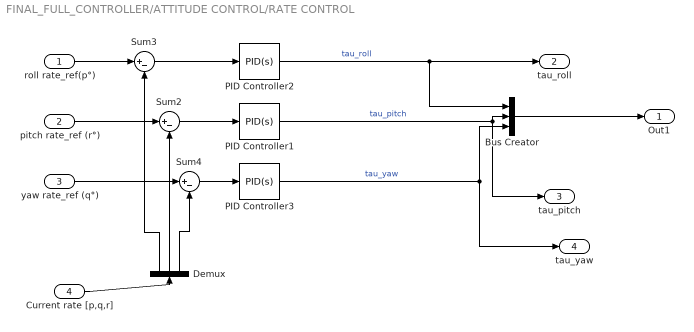
== system FINAL_FULL_CONTROLLER/ATTITUDE CONTROL/RATE CONTROL ==
  " roll rate_ref(p°)" : Inport
  pitch rate_ref (r°) : Inport  Port=2
  yaw rate_ref (q°) : Inport  Port=3
  Current rate [p,q,r] : Inport  Port=4
  Bus Creator : BusCreator  Inputs=3
  Demux : Demux  Outputs=3
  PID Controller1 : slpidlib/PID Controller  Controller=PID  Form=Parallel  TimeDomain=Continuous-time  UseExternalTs=off  SampleTime=-1  IntegratorMethod=Forward Euler  FilterMethod=Forward Euler  ControllerParametersSource=internal  P=0.5549418101336034  I=1.02763096020128  UseKiTs=off  D=-0.000924069987694045  N=73.1912528685867  UseFilter=on  TunerSelectOption=Transfer Function Based (PID Tuner App)  InitialConditionSource=internal  InitialConditionForIntegrator=0  InitialConditionForFilter=0  DifferentiatorICPrevScaledInput=0  ExternalReset=none  TrackingMode=off  Kt=1  LimitOutput=on  SatLimitsSource=internal  UpperSaturationLimit=2*ct*dy*(wmax^2)  LowerSaturationLimit=-2*ct*dy*(wmax^2)  LinearizeAsGain=on  AntiWindupMode=back-calculation  Kb=1  LimitIntegrator=off  UpperIntegratorSaturationLimit=inf  LowerIntegratorSaturationLimit=-inf  POutMin=[]  POutMax=[]  IOutMin=[]  IOutMax=[]  DOutMin=[]  DOutMax=[]  NOutMin=[]  NOutMax=[]  SumOutMin=[]  SumOutMax=[]  SaturationOutMin=[]  SaturationOutMax=[]  PParamMin=[]  PParamMax=[]  IParamMin=[]  IParamMax=[]  DParamMin=[]  DParamMax=[]  NParamMin=[]  NParamMax=[]  KbParamMin=[]  KbParamMax=[]  KtParamMin=[]  KtParamMax=[]  KbOutMin=[]  KbOutMax=[]  KtOutMin=[]  KtOutMax=[]  IntegratorOutMin=[]  IntegratorOutMax=[]  FilterOutMin=[]  FilterOutMax=[]  SumI1OutMin=[]  SumI1OutMax=[]  SumI2OutMin=[]  SumI2OutMax=[]  SumI3OutMin=[]  SumI3OutMax=[]  SumI4OutMin=[]  SumI4OutMax=[]  SumDOutMin=[]  SumDOutMax=[]  DifferentiatorOutMin=[]  DifferentiatorOutMax=[]  FilterDiffOutCoefMin=[]  FilterDiffOutCoefMax=[]  ReciprocalOutMin=[]  ReciprocalOutMax=[]  SumDenOutMin=[]  SumDenOutMax=[]  SumNumOutMin=[]  SumNumOutMax=[]  DivideOutMin=[]  DivideOutMax=[]  UdiffTsProdOutMin=[]  UdiffTsProdOutMax=[]  NTsProdOutMin=[]  NTsProdOutMax=[]  UintegralTsProdOutMin=[]  UintegralTsProdOutMax=[]  UngainTsProdOutMin=[]  UngainTsProdOutMax=[]  ClampingZeroOutDataTypeStr=Inherit: Inherit via back propagation  ClampingZeroOutMin=[]  ClampingZeroOutMax=[]  FilterDenConstantOutDataTypeStr=Inherit: Inherit via back propagation  FilterDenConstantOutMin=[]  FilterDenConstantOutMax=[]  PCopyOutDataTypeStr=Inherit: Inherit via back propagation  PCopyOutMin=[]  PCopyOutMax=[]  NCopyOutDataTypeStr=Inherit: Inherit via back propagation  NCopyOutMin=[]  NCopyOutMax=[]  IntegratorContinuousStateAttributes=''  IntegratorStateMustResolveToSignalObject=off  IntegratorRTWStateStorageClass=Auto  FilterContinuousStateAttributes=''  FilterStateMustResolveToSignalObject=off  FilterRTWStateStorageClass=Auto  ParallelPVariant=InternalParameters  IdealPVariant=Disabled  IVariant=InternalParameters  DVariant=InternalParameters  IntegratorVariant=Continuous  SatVariant=Enabled  AWVariant=BackCalculation  PCopyVariant=Disabled  TRVariant=Disabled  FdbkBlocksVariant=Forward  IdealPFdbkVariant=Disabled  SatFdbkVariant=Disabled  DerivativeFilterVariant=ContFilter  NVariant=InternalParameters  NCopyVariant=Disabled  FilterICVariant=InternalICsFilter  IntegratorICVariant=InternalICs  ExternalResetVariant=Disabled  TRSumVariant=Passthrough  SumFdbkVariant=Disabled  SumVariant=Sum_PID  TsampFilterVariant=InternalTs  TsampNgainVariant=Passthrough  TsampIntegralVariant=Disabled_SignalSpec  ExternalSaturationOutDataTypeStr=Inherit: Same as second input
  PID Controller2 : slpidlib/PID Controller  Controller=PID  Form=Parallel  TimeDomain=Continuous-time  UseExternalTs=off  SampleTime=-1  IntegratorMethod=Forward Euler  FilterMethod=Forward Euler  ControllerParametersSource=internal  P=0.24349143407175  I=1.00321241659327  UseKiTs=off  D=-0.00090211225766007  N=73.1912528649269  UseFilter=on  TunerSelectOption=Transfer Function Based (PID Tuner App)  InitialConditionSource=internal  InitialConditionForIntegrator=0  InitialConditionForFilter=0  DifferentiatorICPrevScaledInput=0  ExternalReset=none  TrackingMode=off  Kt=1  LimitOutput=on  SatLimitsSource=internal  UpperSaturationLimit=2*ct*dx*(wmax^2)  LowerSaturationLimit=-2*ct*dx*(wmax^2)  LinearizeAsGain=on  AntiWindupMode=back-calculation  Kb=1  LimitIntegrator=off  UpperIntegratorSaturationLimit=inf  LowerIntegratorSaturationLimit=-inf  POutMin=[]  POutMax=[]  IOutMin=[]  IOutMax=[]  DOutMin=[]  DOutMax=[]  NOutMin=[]  NOutMax=[]  SumOutMin=[]  SumOutMax=[]  SaturationOutMin=[]  SaturationOutMax=[]  PParamMin=[]  PParamMax=[]  IParamMin=[]  IParamMax=[]  DParamMin=[]  DParamMax=[]  NParamMin=[]  NParamMax=[]  KbParamMin=[]  KbParamMax=[]  KtParamMin=[]  KtParamMax=[]  KbOutMin=[]  KbOutMax=[]  KtOutMin=[]  KtOutMax=[]  IntegratorOutMin=[]  IntegratorOutMax=[]  FilterOutMin=[]  FilterOutMax=[]  SumI1OutMin=[]  SumI1OutMax=[]  SumI2OutMin=[]  SumI2OutMax=[]  SumI3OutMin=[]  SumI3OutMax=[]  SumI4OutMin=[]  SumI4OutMax=[]  SumDOutMin=[]  SumDOutMax=[]  DifferentiatorOutMin=[]  DifferentiatorOutMax=[]  FilterDiffOutCoefMin=[]  FilterDiffOutCoefMax=[]  ReciprocalOutMin=[]  ReciprocalOutMax=[]  SumDenOutMin=[]  SumDenOutMax=[]  SumNumOutMin=[]  SumNumOutMax=[]  DivideOutMin=[]  DivideOutMax=[]  UdiffTsProdOutMin=[]  UdiffTsProdOutMax=[]  NTsProdOutMin=[]  NTsProdOutMax=[]  UintegralTsProdOutMin=[]  UintegralTsProdOutMax=[]  UngainTsProdOutMin=[]  UngainTsProdOutMax=[]  ClampingZeroOutDataTypeStr=Inherit: Inherit via back propagation  ClampingZeroOutMin=[]  ClampingZeroOutMax=[]  FilterDenConstantOutDataTypeStr=Inherit: Inherit via back propagation  FilterDenConstantOutMin=[]  FilterDenConstantOutMax=[]  PCopyOutDataTypeStr=Inherit: Inherit via back propagation  PCopyOutMin=[]  PCopyOutMax=[]  NCopyOutDataTypeStr=Inherit: Inherit via back propagation  NCopyOutMin=[]  NCopyOutMax=[]  IntegratorContinuousStateAttributes=''  IntegratorStateMustResolveToSignalObject=off  IntegratorRTWStateStorageClass=Auto  FilterContinuousStateAttributes=''  FilterStateMustResolveToSignalObject=off  FilterRTWStateStorageClass=Auto  ParallelPVariant=InternalParameters  IdealPVariant=Disabled  IVariant=InternalParameters  DVariant=InternalParameters  IntegratorVariant=Continuous  SatVariant=Enabled  AWVariant=BackCalculation  PCopyVariant=Disabled  TRVariant=Disabled  FdbkBlocksVariant=Forward  IdealPFdbkVariant=Disabled  SatFdbkVariant=Disabled  DerivativeFilterVariant=ContFilter  NVariant=InternalParameters  NCopyVariant=Disabled  FilterICVariant=InternalICsFilter  IntegratorICVariant=InternalICs  ExternalResetVariant=Disabled  TRSumVariant=Passthrough  SumFdbkVariant=Disabled  SumVariant=Sum_PID  TsampFilterVariant=InternalTs  TsampNgainVariant=Passthrough  TsampIntegralVariant=Disabled_SignalSpec  ExternalSaturationOutDataTypeStr=Inherit: Same as second input
  PID Controller3 : slpidlib/PID Controller  Controller=PID  Form=Parallel  TimeDomain=Continuous-time  UseExternalTs=off  SampleTime=-1  IntegratorMethod=Forward Euler  FilterMethod=Forward Euler  ControllerParametersSource=internal  P=0.577394225548127  I=0.730884395914263  UseKiTs=off  D=-0.00065722848080941  N=73.1912528649269  UseFilter=on  TunerSelectOption=Transfer Function Based (PID Tuner App)  InitialConditionSource=internal  InitialConditionForIntegrator=0  InitialConditionForFilter=0  DifferentiatorICPrevScaledInput=0  ExternalReset=none  TrackingMode=off  Kt=1  LimitOutput=on  SatLimitsSource=internal  UpperSaturationLimit=-inv(I(3,3))*(2*cq*wmax^2)  LowerSaturationLimit=inv(I(3,3))*(2*cq*wmax^2)  LinearizeAsGain=on  AntiWindupMode=back-calculation  Kb=3  LimitIntegrator=off  UpperIntegratorSaturationLimit=inf  LowerIntegratorSaturationLimit=-inf  POutMin=[]  POutMax=[]  IOutMin=[]  IOutMax=[]  DOutMin=[]  DOutMax=[]  NOutMin=[]  NOutMax=[]  SumOutMin=[]  SumOutMax=[]  SaturationOutMin=[]  SaturationOutMax=[]  PParamMin=[]  PParamMax=[]  IParamMin=[]  IParamMax=[]  DParamMin=[]  DParamMax=[]  NParamMin=[]  NParamMax=[]  KbParamMin=[]  KbParamMax=[]  KtParamMin=[]  KtParamMax=[]  KbOutMin=[]  KbOutMax=[]  KtOutMin=[]  KtOutMax=[]  IntegratorOutMin=[]  IntegratorOutMax=[]  FilterOutMin=[]  FilterOutMax=[]  SumI1OutMin=[]  SumI1OutMax=[]  SumI2OutMin=[]  SumI2OutMax=[]  SumI3OutMin=[]  SumI3OutMax=[]  SumI4OutMin=[]  SumI4OutMax=[]  SumDOutMin=[]  SumDOutMax=[]  DifferentiatorOutMin=[]  DifferentiatorOutMax=[]  FilterDiffOutCoefMin=[]  FilterDiffOutCoefMax=[]  ReciprocalOutMin=[]  ReciprocalOutMax=[]  SumDenOutMin=[]  SumDenOutMax=[]  SumNumOutMin=[]  SumNumOutMax=[]  DivideOutMin=[]  DivideOutMax=[]  UdiffTsProdOutMin=[]  UdiffTsProdOutMax=[]  NTsProdOutMin=[]  NTsProdOutMax=[]  UintegralTsProdOutMin=[]  UintegralTsProdOutMax=[]  UngainTsProdOutMin=[]  UngainTsProdOutMax=[]  ClampingZeroOutDataTypeStr=Inherit: Inherit via back propagation  ClampingZeroOutMin=[]  ClampingZeroOutMax=[]  FilterDenConstantOutDataTypeStr=Inherit: Inherit via back propagation  FilterDenConstantOutMin=[]  FilterDenConstantOutMax=[]  PCopyOutDataTypeStr=Inherit: Inherit via back propagation  PCopyOutMin=[]  PCopyOutMax=[]  NCopyOutDataTypeStr=Inherit: Inherit via back propagation  NCopyOutMin=[]  NCopyOutMax=[]  IntegratorContinuousStateAttributes=''  IntegratorStateMustResolveToSignalObject=off  IntegratorRTWStateStorageClass=Auto  FilterContinuousStateAttributes=''  FilterStateMustResolveToSignalObject=off  FilterRTWStateStorageClass=Auto  ParallelPVariant=InternalParameters  IdealPVariant=Disabled  IVariant=InternalParameters  DVariant=InternalParameters  IntegratorVariant=Continuous  SatVariant=Enabled  AWVariant=BackCalculation  PCopyVariant=Disabled  TRVariant=Disabled  FdbkBlocksVariant=Forward  IdealPFdbkVariant=Disabled  SatFdbkVariant=Disabled  DerivativeFilterVariant=ContFilter  NVariant=InternalParameters  NCopyVariant=Disabled  FilterICVariant=InternalICsFilter  IntegratorICVariant=InternalICs  ExternalResetVariant=Disabled  TRSumVariant=Passthrough  SumFdbkVariant=Disabled  SumVariant=Sum_PID  TsampFilterVariant=InternalTs  TsampNgainVariant=Passthrough  TsampIntegralVariant=Disabled_SignalSpec  ExternalSaturationOutDataTypeStr=Inherit: Same as second input
  Sum2 : Sum  Inputs=|+-
  Sum3 : Sum  Inputs=|+-
  Sum4 : Sum  Inputs=|+-
  Out1 : Outport
  tau_roll : Outport  Port=2
  tau_pitch : Outport  Port=3
  tau_yaw : Outport  Port=4
  wires:
  PID Controller3/1 -> Bus Creator/3, tau_yaw/1  "tau_yaw"
  Demux/3 -> Sum4/2
  Sum2/1 -> PID Controller1/1
  Sum4/1 -> PID Controller3/1
  PID Controller1/1 -> Bus Creator/2, tau_pitch/1  "tau_pitch"
  " roll rate_ref(p°)"/1 -> Sum3/1
  Demux/1 -> Sum3/2
  Demux/2 -> Sum2/2
  Current rate [p,q,r]/1 -> Demux/1
  pitch rate_ref (r°)/1 -> Sum2/1
  yaw rate_ref (q°)/1 -> Sum4/1
  PID Controller2/1 -> Bus Creator/1, tau_roll/1  "tau_roll"
  Sum3/1 -> PID Controller2/1
  Bus Creator/1 -> Out1/1

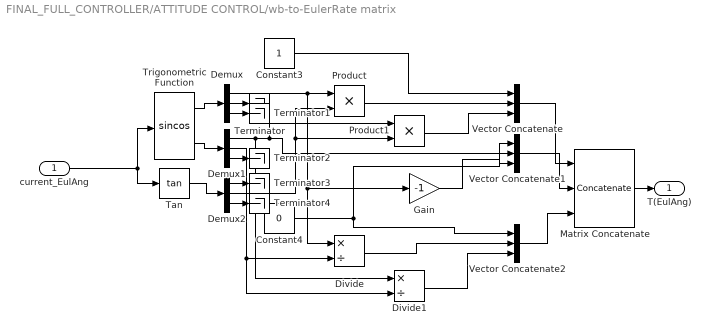
== system FINAL_FULL_CONTROLLER/ATTITUDE CONTROL/wb-to-EulerRate matrix ==
  current_EulAng : Inport
  Constant3 : Constant
  Constant4 : Constant  Value=0
  Demux : Demux  Outputs=3
  Demux1 : Demux  Outputs=3
  Demux2 : Demux  Outputs=3
  Divide : Product  Inputs=*/
  Divide1 : Product  Inputs=*/
  Gain : Gain  Gain=-1
  Matrix Concatenate : Concatenate  NumInputs=3  Mode=Multidimensional array
  Product : Product
  Product1 : Product
  Tan : Trigonometry  Operator=tan
  Terminator{,1..4} (5 alike) : Terminator
  Trigonometric Function : Trigonometry  Operator=sincos
  Vector Concatenate : Concatenate  NumInputs=3  Mode=Multidimensional array  ConcatenateDimension=2
  Vector Concatenate1 : Concatenate  NumInputs=3  Mode=Multidimensional array  ConcatenateDimension=2
  Vector Concatenate2 : Concatenate  NumInputs=3  Mode=Multidimensional array  ConcatenateDimension=2
  T(EulAng) : Outport
  wires:
  Demux1/1 -> Divide1/1, Vector Concatenate1/2, Product1/1
  Demux/1 -> Divide/1, Gain/1, Product/1
  Matrix Concatenate/1 -> T(EulAng)/1
  Demux2/2 -> Product1/2, Product/2
  Divide/1 -> Vector Concatenate2/2
  Product/1 -> Vector Concatenate/2
  Vector Concatenate/1 -> Matrix Concatenate/1
  current_EulAng/1 -> Trigonometric Function/1, Tan/1
  Constant3/1 -> Vector Concatenate/1
  Demux/2 -> Terminator/1
  Trigonometric Function/2 -> Demux1/1
  Constant4/1 -> Vector Concatenate2/1, Vector Concatenate1/1
  Vector Concatenate2/1 -> Matrix Concatenate/3
  Demux1/3 -> Terminator2/1
  Demux1/2 -> Divide1/2, Divide/2
  Product1/1 -> Vector Concatenate/3
  Divide1/1 -> Vector Concatenate2/3
  Vector Concatenate1/1 -> Matrix Concatenate/2
  Trigonometric Function/1 -> Demux/1
  Gain/1 -> Vector Concatenate1/3
  Tan/1 -> Demux2/1
  Demux/3 -> Terminator1/1
  Demux2/1 -> Terminator3/1
  Demux2/3 -> Terminator4/1

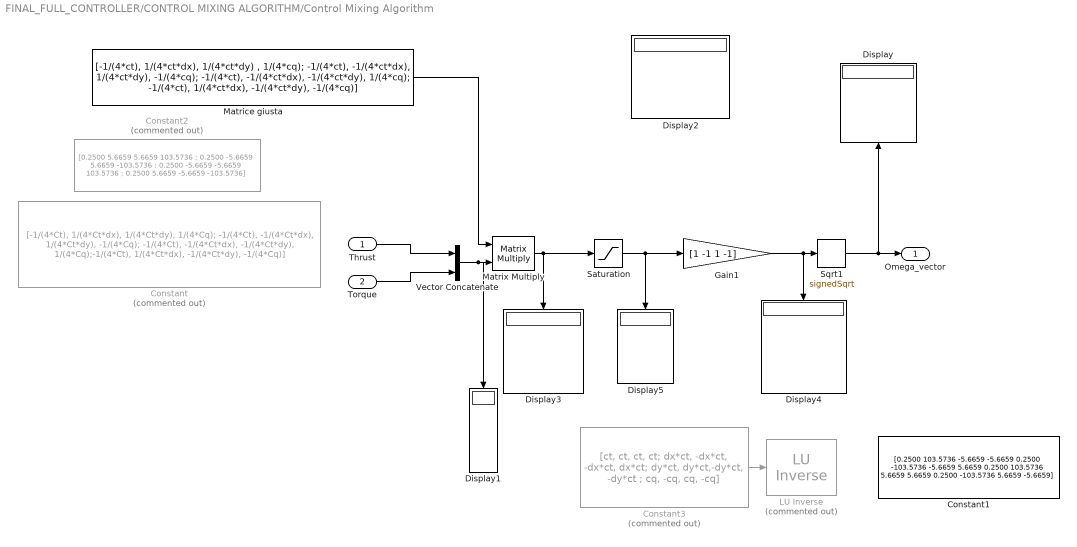
== system FINAL_FULL_CONTROLLER/CONTROL MIXING ALGORITHM/Control Mixing Algorithm ==
  Thrust : Inport
  Torque : Inport  Port=2
  " LU Inverse" : dspinverses/ LU Inverse  Commented=on
  Constant : Constant  Commented=on  Value="[-1/(4*Ct),  1/(4*Ct*dx),  1/(4*Ct*dy),  1/(4*Cq); -1/(4*Ct), -1/(4*Ct*dx),  1/(4*Ct*dy), -1/(4*Cq); -1/(4*Ct), -1/(4*Ct*dx), -1/(4*Ct*dy),  1/(4*Cq);-1/(4*Ct),  1/(4*Ct*dx), -1/(4*Ct*dy), -1/(4*Cq)]"
  Constant1 : Constant  Value=|
      | [0.2500  103.5736   -5.6659   -5.6659
      |     0.2500 -103.5736   -5.6659    5.6659
      |     0.2500  103.5736    5.6659    5.6659
      |     0.2500 -103.5736    5.6659   -5.6659]
  Constant2 : Constant  Commented=on  Value=|  VectorParams1D=off
      | [0.2500    5.6659    5.6659  103.5736
      | ;    0.2500   -5.6659    5.6659 -103.5736
      |   ;  0.2500   -5.6659   -5.6659  103.5736
      |  ;   0.2500    5.6659   -5.6659 -103.5736]
  Constant3 : Constant  Commented=on  Value=[ct, ct, ct, ct; dx*ct, -dx*ct, -dx*ct, dx*ct; dy*ct, dy*ct,-dy*ct, -dy*ct ; cq, -cq, cq, -cq]
  Display{,1..5} (6 alike) : Display
  Gain1 : Gain  Gain=[1 -1 1 -1]
  Matrice giusta : Constant  Value="[-1/(4*ct), 1/(4*ct*dx), 1/(4*ct*dy) ,  1/(4*cq); -1/(4*ct),  -1/(4*ct*dx), 1/(4*ct*dy), -1/(4*cq); -1/(4*ct),  -1/(4*ct*dx),  -1/(4*ct*dy),  1/(4*cq); -1/(4*ct), 1/(4*ct*dx),  -1/(4*ct*dy), -1/(4*cq)]"  VectorParams1D=off
  Matrix Multiply : Product  Multiplication=Matrix(*)
  Saturation : Saturate  UpperLimit=inf  LowerLimit=0
  Sqrt1 : Sqrt  Operator=signedSqrt
  Vector Concatenate : Concatenate
  Omega_vector : Outport
  wires:
  Constant3/1 -> " LU Inverse"/1
  Thrust/1 -> Vector Concatenate/1
  Torque/1 -> Vector Concatenate/2
  Sqrt1/1 -> Display/1, Omega_vector/1
  Matrice giusta/1 -> Matrix Multiply/1
  Vector Concatenate/1 -> Display1/1, Matrix Multiply/2
  Gain1/1 -> Display4/1, Sqrt1/1
  Matrix Multiply/1 -> Saturation/1, Display3/1
  Saturation/1 -> Gain1/1, Display5/1

== system FINAL_FULL_CONTROLLER/AIRFRAME/6DoF Model in a  gravity field/Gravità_modello ==
  DCM_be : Inport
  Change of reference system1 : Product  Multiplication=Matrix(*)
  gravity force(f) : Constant  Value=[0,0,g*(4*m+m1+m2+m3+m4)]'
  Gravità : Outport
  wires:
  gravity force(f)/1 -> Change of reference system1/2
  Change of reference system1/1 -> Gravità/1  "gravity in terna body"
  DCM_be/1 -> Change of reference system1/1
